simulink model "Manipulator_PDControl_AdaptiveInverseDynamics"  (R2020b)
settings: Solver=FixedStepAuto  StartTime=0.0  StopTime=t_final  FixedStep=dt  RelTol=1e-3
values from neighbouring files (symbols this model uses):
  dq_0 = 0.1 *[ 0  -1  0]    [Initialization.m]
  dt = 1.00e-03    (= 0.001)    [Initialization.m]
  ikInitGuessSim = ikInitGuess    [generateTrajectory.m]
  P = lyap(A',Q)    [robustInvDynamicsInit.m]    (also in robustInverseDyn.m)
  q_0 = [0;-0.9;2.7]    [Initialization.m]
  theta_params_init = [p1; p2 ... (first row only)    [AdaptiveInverseDynamicsInit.m]
  waypointAccels = zeros(size(waypointVels))    [generateTrajectory.m]
  waypoints = initPosition +              [0 0 0 ; 0 -a -a ; 0 0 -2*a; 0 a -a ; 0 0 0]'    [generateTrajectory.m]
  waypointVels = 0.1 *[ 0  -1  0 ... (first row only)    [generateTrajectory.m]
libraries: simulink x3, robotcorelib x2, robotmaniplib x1
settings Model: Creator=m2aali  LastModifiedBy=Kons
settings DataIOCC: LoggingToFile=on

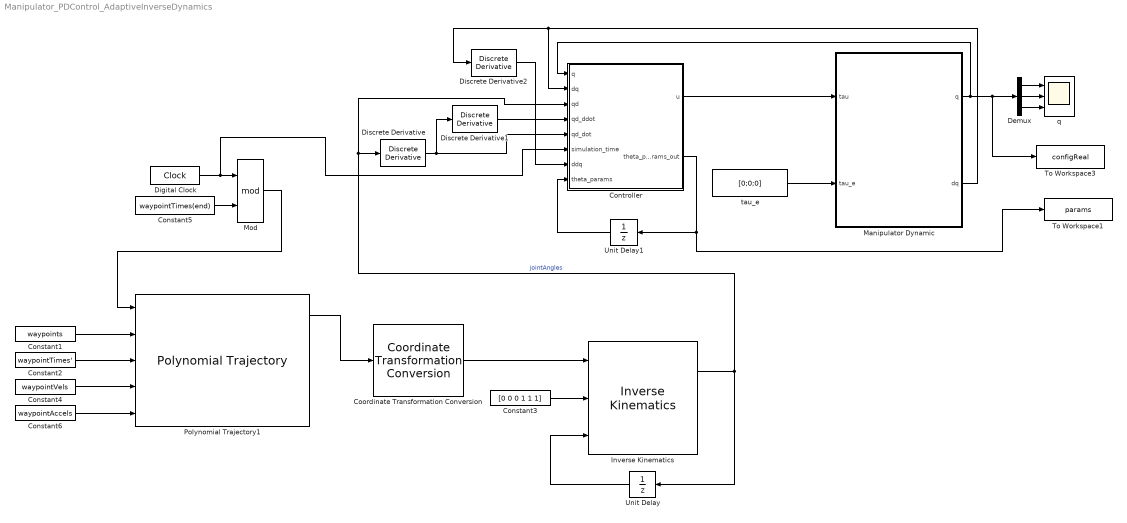
== system Manipulator_PDControl_AdaptiveInverseDynamics ==
  Constant1 : Constant  Value=waypoints  VectorParams1D=off  SampleTime=-1
  Constant2 : Constant  Value=waypointTimes'  VectorParams1D=off  SampleTime=-1
  Constant3 : Constant  Value=[0 0 0 1 1 1]  VectorParams1D=off
  Constant4 : Constant  Value=waypointVels  VectorParams1D=off  SampleTime=-1
  Constant5 : Constant  Value=waypointTimes(end)
  Constant6 : Constant  Value=waypointAccels  VectorParams1D=off  SampleTime=-1
  Controller : Subsystem
  Coordinate Transformation Conversion : robotcorelib/Coordinate Transformation Conversion  InputRepresentation=Translation Vector  InputEulerSequence=ZYX  ShowTrVecInputPort=on  OutputRepresentation=Homogeneous Transformation  OutputEulerSequence=ZYX  ShowTrVecOutputPort=on  SimulateUsing=Code generation
      settings: SourceProductBaseCode=NV,RO,RR,UV
  Demux : Demux  Outputs=3
  Digital Clock : DigitalClock  SampleTime=dt
  Discrete Derivative : simulink/Discrete/Discrete Derivative  gainval=1.0  ICPrevScaledInput=[-0.000001274337461;-0.900000000000479;2.699999999999876]*1000  OutMin=[]  OutMax=[]  OutDataType=fixdt(1, 16)  OutScaling=2^-10  DoSatur=off
  Discrete Derivative1 : simulink/Discrete/Discrete Derivative  gainval=1.0  ICPrevScaledInput="[ 0 ; 0;  0]"  OutMin=[]  OutMax=[]  OutDataType=fixdt(1, 16)  OutScaling=2^-10  DoSatur=off
  Discrete Derivative2 : simulink/Discrete/Discrete Derivative  gainval=1.0  ICPrevScaledInput="[ 0 ; 0;  0]"  OutMin=[]  OutMax=[]  OutDataType=fixdt(1, 16)  OutScaling=2^-10  DoSatur=off
  Inverse Kinematics : robotmaniplib/Inverse Kinematics  RigidBodyTree=robot  EndEffector=Link_EE  ShowInfo=on  SolverName=BFGS Gradient Projection  EnforceJointLimits=on  MaxIterations=1500  MaxTime=10  GradientTolerance=1e-7  SolutionTolerance=1e-6  StepTolerance=1e-14  ErrorChangeTolerance=1e-12  UseErrorDamping=on  DampingBias=0.0025  SimulateUsing=Code generation
  Manipulator Dynamic : Subsystem
  Mod : Math  Operator=mod  SignedPower=on  SaturateOnIntegerOverflow=on
  Polynomial Trajectory1 : robotcorelib/Polynomial Trajectory  WaypointSource=External  Waypoints=[ 0, 2, 1, 5, 0; -1, 3, 1, 4, 4 ]  TimePoints=[ 0, 1, 2, 3, 4 ]  TimeInterval=[ 1, 4 ]  Method=Quintic Polynomial  ParameterSource=External  VelocityBoundaryCondition=zeros( 2, 5 )  AccelerationBoundaryCondition=zeros( 2, 5 )  SimulateUsing=Code generation
  To Workspace1 : ToWorkspace  VariableName=params  SaveFormat=Timeseries  SampleTime=-1
  To Workspace3 : ToWorkspace  VariableName=configReal  SaveFormat=Timeseries  SampleTime=-1
  Unit Delay : UnitDelay  InitialCondition=ikInitGuessSim  SampleTime=-1  HasFrameUpgradeWarning=on
  Unit Delay1 : UnitDelay  InitialCondition=theta_params_init  SampleTime=-1  HasFrameUpgradeWarning=on
  q : Scope  NumInputPorts=3
  tau_e : Constant  Value=[0;0;0]
  wires:
  tau_e/1 -> Manipulator Dynamic/2(tau_e)
  Manipulator Dynamic/2(dq) -> Discrete Derivative2/1, Controller/2(dq)
  Controller/1(u) -> Manipulator Dynamic/1(tau)
  Demux/1 -> q/1
  Demux/2 -> q/2
  Demux/3 -> q/3
  Digital Clock/1 -> Controller/6(simulation_time), Mod/1
  Mod/1 -> Polynomial Trajectory1/1
  Constant5/1 -> Mod/2
  Polynomial Trajectory1/1 -> Coordinate Transformation Conversion/1
  Inverse Kinematics/1 -> Unit Delay/1, Controller/3(qd), Discrete Derivative/1  "jointAngles"
  Unit Delay/1 -> Inverse Kinematics/3
  Constant3/1 -> Inverse Kinematics/2
  Coordinate Transformation Conversion/1 -> Inverse Kinematics/1
  Discrete Derivative1/1 -> Controller/4(qd_ddot)
  Discrete Derivative/1 -> Discrete Derivative1/1, Controller/5(qd_dot)
  Constant1/1 -> Polynomial Trajectory1/2
  Constant2/1 -> Polynomial Trajectory1/3
  Constant4/1 -> Polynomial Trajectory1/4
  Constant6/1 -> Polynomial Trajectory1/5
  Manipulator Dynamic/1(q) -> To Workspace3/1, Demux/1, Controller/1(q)
  Discrete Derivative2/1 -> Controller/7(ddq)
  Controller/2(theta_params_out) -> To Workspace1/1, Unit Delay1/1
  Unit Delay1/1 -> Controller/8(theta_params)

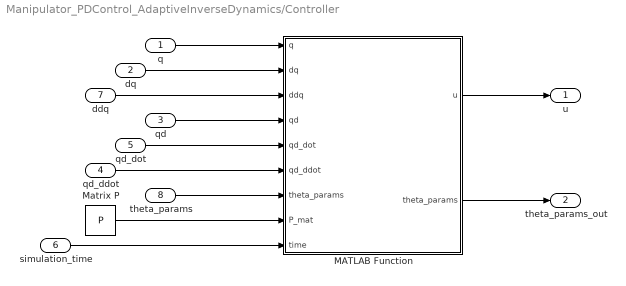
== system Manipulator_PDControl_AdaptiveInverseDynamics/Controller ==
  q : Inport
  dq : Inport  Port=2
  qd : Inport  Port=3
  qd_ddot : Inport  Port=4
  qd_dot : Inport  Port=5
  simulation_time : Inport  Port=6
  ddq : Inport  Port=7
  theta_params : Inport  Port=8
  MATLAB Function : MATLAB Function  TreatAsAtomicUnit=on
  Matrix P : Constant  Value=P
  u : Outport
  theta_params_out : Outport  Port=2
  wires:
  dq/1 -> MATLAB Function/2(dq)
  MATLAB Function/1(u) -> u/1
  qd/1 -> MATLAB Function/4(qd)
  q/1 -> MATLAB Function/1(q)
  qd_ddot/1 -> MATLAB Function/6(qd_ddot)
  qd_dot/1 -> MATLAB Function/5(qd_dot)
  simulation_time/1 -> MATLAB Function/9(time)
  Matrix P/1 -> MATLAB Function/8(P_mat)
  ddq/1 -> MATLAB Function/3(ddq)
  theta_params/1 -> MATLAB Function/7("theta_params ")
  MATLAB Function/2(theta_params) -> theta_params_out/1

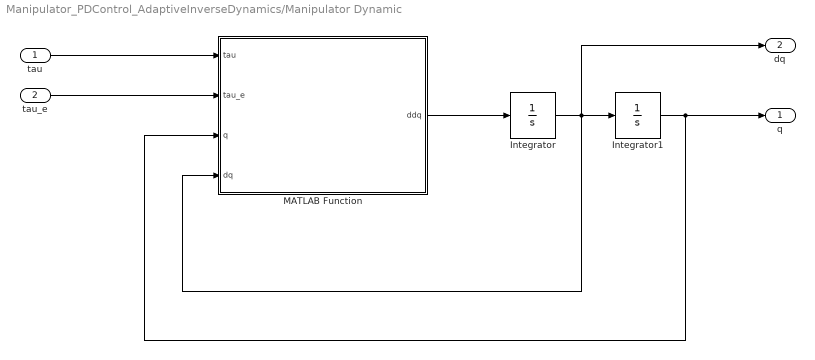
== system Manipulator_PDControl_AdaptiveInverseDynamics/Manipulator Dynamic ==
  tau : Inport
  tau_e : Inport  Port=2
  Integrator : Integrator  InitialCondition=dq_0
  Integrator1 : Integrator  InitialCondition=q_0
  MATLAB Function : MATLAB Function  TreatAsAtomicUnit=on
  q : Outport
  dq : Outport  Port=2
  wires:
  MATLAB Function/1(ddq) -> Integrator/1
  tau/1 -> MATLAB Function/1(tau)
  tau_e/1 -> MATLAB Function/2(tau_e)
  Integrator1/1 -> q/1, MATLAB Function/3(q)
  Integrator/1 -> dq/1, MATLAB Function/4(dq), Integrator1/1

== matlab function Manipulator_PDControl_AdaptiveInverseDynamics/Controller/MATLAB Function ==
  data: q input; dq input; ddq input; u output; qd input; qd_dot input; qd_ddot input; theta_params input; P_mat input; time input; theta_params output
function [u, theta_params] = fcn(q, dq, ddq, qd, qd_dot, qd_ddot, theta_params,...
                                                                  P_mat, time)
% PD + gravity compensation controller function

%% reset first qd_ddot
if (time < 0.003)
    qd_ddot = [0;0;0];
    qd_dot = [0;0;0];
    ddq = [0;0;0];
end

%% PD Controller Parameters 
Kp = [2,0,0; 0, 2 ,0; 0, 0 , 2];  %  Kp is 3*3 matrix of proportional gain 
Kd = [5,0,0; 0, 5 ,0; 0, 0 , 5]; %Kd is 3*3 matrix of derivative gain

%% calculate aq

aq = qd_ddot - Kp * (q - qd) - Kd * (dq - qd_dot);

%% calculate control 

u = getRegressorY(q,dq,aq) * theta_params;

%% calculate H_hat

H_hat = getHEstimate(q, theta_params);
H = getH(q);
%% parameter adaptation algorithm

G_matrix = diag([1,1,1,1,1,1,1,1])/10;
Fi_matrix = inv(H) * getRegressorY(q,dq,ddq);
error = [q - qd; dq - qd_dot];

%% define B
zrs = zeros(3);
I = eye(3);
B = [zrs;I];

%% get theta derivative
dTheta_params = -inv(G_matrix)*Fi_matrix'*(B'*P_mat*error);
% Fi_matrix = inv(H_hat) * getRegressorY(q,dq,ddq)   3x3  x   3x8 =   3x8
% G 8x8, fi' 8x3 === 8x3
% -inv(G_matrix)*Fi_matrix' 8x3
% B' 1x6
% P_mat 6x6
% error 6x1
% P_mat*error 6x1
% B'*P_mat*error = 1x1

% Y = getRegressorY(q,dq,ddq);
% dTheta_params = -inv(G_matrix) * Y' * inv(H_hat) * B' * P_mat*error;

%% update theta params
dt = 0.001;
theta_params = theta_params + dTheta_params*dt;

% dynReg = getRegressorY(q,dq,ddq) * theta_params;
% dynOrd = H_hat*ddq + C_hat*dq + G_hat;

%% define regressor Y

function [Y] = getRegressorY(q,dq,ddq)
q1 = q(1);
q2 = q(2);
q3 = q(3);

dq1 = dq(1);
dq2 = dq(2);
dq3 = dq(3);

ddq1 = ddq(1);
ddq2 = ddq(2);
ddq3 = ddq(3);

c2 = cos(q2);
s23 = sin(q2 + q3);
c23 = cos(q2+q3);
s3 = sin(q3);
c3 = cos(q3);
%% 1 row
H_1row = ddq1 * [1,   c2^2,    c2^2,     s23^2, 2*c2*s23,0,0,0];
C_1row_1part = dq1 * dq2 * [0,  -sin(2*q2),  -sin(2*q2), sin(2*(q1+q2)), ...
                2*cos(2*q2+q3), 0,  0,  0];
C_1row_2part = dq3 * dq3 * [0, 0, 0, sin(2*(q2+q3)), 2*c2*c23, 0,0,0];
C_1row = C_1row_1part + C_1row_2part;

Y_1row = H_1row + C_1row;

%% 2 row
H_2row_1part = ddq2 * [0, 1,1,1,2*s3,0,0,0];
H_2row_2part = ddq3 * [0,0,0,1,s3,0,0,0];
H_2row = H_2row_1part + H_2row_2part;

C_2row_1part = dq1 * dq1 * (1/2) * [0, sin(2*q2),sin(2*q2), -sin(2*(q2+q3)), ...
                                -2*cos(2*q2+q3),0,0,0];
C_2row_2part = dq3 * [0,0,0,0,  2*c3*dq2 + c3*dq3,  0,0,0];
C_2row = C_2row_1part + C_2row_2part;

G_2row = [0,0,0,0,0, -c2,-c2,-s23];

Y_2row = H_2row + C_2row + G_2row;

%% 3 row
H_3row_1part = ddq2 * [0,0,0,1,s3,0,0,0];
H_3row_2part = ddq3 * [0,0,0,1,0,0,0,0];
H_3row = H_3row_1part + H_3row_2part;

C_3row_1part = -(1/2) * dq1 * dq1 * [0,0,0, sin(2*(q2+q3)), c2*c23,0,0,0];
C_3row_2part = dq2 * dq2 * [0,0,0,0,-c3*dq2, 0,0,0];
C_3row = C_3row_1part + C_3row_2part;

G_3row = [0,0,0,0,0,0,0,-s23];

Y_3row = H_3row + C_3row + G_3row;

%% Y
Y = [Y_1row; 
     Y_2row;
     Y_3row];

%% get H estimate
function [H_hat] = getHEstimate(q, theta_params)

q1 = q(1);
q2 = q(2);
q3 = q(3);

p1 = theta_params(1);
p2 = theta_params(2);
p3 = theta_params(3);
p4 = theta_params(4);
p5 = theta_params(5);

J_hat = p1;
J1 = p4;
J12 = p2 + p3;
J13 = p5;

h11 = J_hat + J1 * (sin(q2 + q3))^2 + J12 * (cos(q2))^2 + 2 * J13 * cos(q2) * sin(q2+q3);
h22 = J1 + J12 + 2 * J13 * sin(q3);
h23 = J1 + J13 * sin(q3);
h32 = h23;
h33 = J1;

H_hat = [h11, 0 ,0 ;
    0 , h22, h23;
    0 , h32, h33];

function [H] = getH(q)
    q1 = q(1);
    q2 = q(2);
    q3 = q(3);

    %% general physical parameters

    l1 = 0.6731;
    l2 = 0.432;
    l3 = 0.434;
    lc2 = 0.216;
    lc3 = 0.164;
    m2 = 15.46;
    m3 = 9.55;
    J = 0.302;

    %% Inertia Matrix Parameters

    J1 = m3 * lc3^2;
    J12 = (m2 * lc2^2) + (m3 * l2^2);
    J13 = l2 * lc3 * m3;


    h11 = J + J1 * (sin(q2 + q3))^2 + J12 * (cos(q2))^2 + 2 * J13 * cos(q2) * sin(q2+q3);
    h22 = J1 + J12 + 2 * J13 * sin(q3);
    h23 = J1 + J13 * sin(q3);
    h32 = h23;
    h33 = J1;

    H = [h11, 0 ,0 ;
        0 , h22, h23;
        0 , h32, h33];

== matlab function Manipulator_PDControl_AdaptiveInverseDynamics/Manipulator Dynamic/MATLAB Function ==
  data: tau input; tau_e input; q input; ddq output; dq input
function ddq = DynamicModel( tau, tau_e, q, dq)
%%%%%
% 3-DOF Puma-560 Dynamic Model Function
% H(q)* ddq + C(q) * dq + G = tau + tau_e
% q is 3*1 vector of joint variables (radian)
% H(q) is the inertia matrix
% C(q) is the matrix of Coriolis and centrifugal forces
% G(q) is  the vector of potential forces Parameters
% tau is control torque 
% tau_e is the external torque due to the interaction with the environment
%%%%%

%% Joint Space variables

q1 = q(1);
q2 = q(2);
q3 = q(3);

dq1 = dq(1);
dq2 = dq(2);
dq3 = dq(3);

%% general physical parameters

l1 = 0.6731;
l2 = 0.432;
l3 = 0.434;
lc2 = 0.216;
lc3 = 0.164;
m2 = 15.46;
m3 = 9.55;
J = 0.302;

%% Inertia Matrix Parameters

J1 = m3 * lc3^2;
J12 = (m2 * lc2^2) + (m3 * l2^2);
J13 = l2 * lc3 * m3;


h11 = J + J1 * (sin(q2 + q3))^2 + J12 * (cos(q2))^2 + 2 * J13 * cos(q2) * sin(q2+q3);
h22 = J1 + J12 + 2 * J13 * sin(q3);
h23 = J1 + J13 * sin(q3);
h32 = h23;
h33 = J1;

H = [h11, 0 ,0 ;
    0 , h22, h23;
    0 , h32, h33];

%% Coriolis Matrix Parameters

c12_1 = J1 * sin(2 * (q1 + q2)) - J12 * sin(2 * q2) + 2 * J13 * cos(2 * q2 +q3);
c13_1 = J1 * sin(2 * (q2 + q3)) + 2 * J13 * cos(q2) * cos(q2 + q3);
c11_2 = (1/2) * (-J1 * sin(2 * (q2 + q3)) + J12 * sin(2 * q2) - 2 * J13 * cos(2 * q2 + q3));
c22_2 = 2 * J13 * cos(q3);
c23_2 = J13 * cos(q3);
c22_3 = -J13 * cos(q3) * dq2;
c11_3 = (-1/2) * (J1 * sin(2 * (q2 + q3)) + J13 * cos(q2) * cos(q2 + q3));

C = [0, c12_1 * dq1, c13_1 * dq3;
    c11_2 * dq1, 0 , c22_2 * dq2 + c23_2 * dq3;
    c11_3 * dq1, c22_3 * dq2, 0];

%% Vector of Potential Forces Parameters

g = 9.81;

g21 = -g * (lc3 * m3 * sin(q2 + q3) + lc2 * m2 * cos(q2) + l2 * m3 * cos(q2));
g31 = -g * (lc3 * m3 * sin(q2 + q3));

G = [0;
    g21;
    g31];

%% Function output

ddq = inv(H)*(tau + tau_e - C * dq - G);
